simulink model "BodyModel_Simulink"  (R2020b)
settings: Solver=ode23tb  StartTime=0.0  StopTime=300  RelTol=1e-3
model workspace (MAT data in the model file):
  A_m = [-1000000  0  0  0  0  0  0  0  0  0  0  0; 0  -1000000  0  0  0  0  0  0  0  0  0  0; 0  0  -1000000  0  0  0  0  0  0  0  0  0; 0  0  0  -1000000  0  0  0  0  0  0  0  0; 0  0  0  0  -1000000  0  0  0  0  0  0  0; 0  0  0  0  0  -1000000  0  0  0  0  0  0; 0  0  0  0  0  0  -1000000  0  0  0  0  0; 0  0  0  0  0  0  0  -1000000  0  0  0  0; 0  0  0  0  0  0  0  0  -1000000  0  0  0; 0  0  0  0  0  0  0  0  0  -1000000  0  0; 0  0  0  0  0  0  0  0  0  0  -1000000  0; 0  0  0  0  0  0  0  0  0  0  0  -1000000]
  B_m = [1000000  0  0  0  0  0  0  0  0  0  0  0; 0  1000000  0  0  0  0  0  0  0  0  0  0; 0  0  1000000  0  0  0  0  0  0  0  0  0; 0  0  0  1000000  0  0  0  0  0  0  0  0; 0  0  0  0  1000000  0  0  0  0  0  0  0; 0  0  0  0  0  1000000  0  0  0  0  0  0; 0  0  0  0  0  0  1000000  0  0  0  0  0; 0  0  0  0  0  0  0  1000000  0  0  0  0; 0  0  0  0  0  0  0  0  1000000  0  0  0; 0  0  0  0  0  0  0  0  0  1000000  0  0; 0  0  0  0  0  0  0  0  0  0  1000000  0; 0  0  0  0  0  0  0  0  0  0  0  1000000]
  C_m = [1  0  0  0  0  0  0  0  0  0  0  0; 0  1  0  0  0  0  0  0  0  0  0  0; 0  0  1  0  0  0  0  0  0  0  0  0; 0  0  0  1  0  0  0  0  0  0  0  0; 0  0  0  0  1  0  0  0  0  0  0  0; 0  0  0  0  0  1  0  0  0  0  0  0; 0  0  0  0  0  0  1  0  0  0  0  0; 0  0  0  0  0  0  0  1  0  0  0  0; 0  0  0  0  0  0  0  0  1  0  0  0; 0  0  0  0  0  0  0  0  0  1  0  0; 0  0  0  0  0  0  0  0  0  0  1  0; 0  0  0  0  0  0  0  0  0  0  0  1]
  D_m = [0  0  0  0  0  0  0  0  0  0  0  0; 0  0  0  0  0  0  0  0  0  0  0  0; 0  0  0  0  0  0  0  0  0  0  0  0; 0  0  0  0  0  0  0  0  0  0  0  0; 0  0  0  0  0  0  0  0  0  0  0  0; 0  0  0  0  0  0  0  0  0  0  0  0; 0  0  0  0  0  0  0  0  0  0  0  0; 0  0  0  0  0  0  0  0  0  0  0  0; 0  0  0  0  0  0  0  0  0  0  0  0; 0  0  0  0  0  0  0  0  0  0  0  0; 0  0  0  0  0  0  0  0  0  0  0  0; 0  0  0  0  0  0  0  0  0  0  0  0]
  K_lqr = [0.500001142903  -0.499931060878  -0.5  1.16845749322  -1.17239239615  -5.45970154425  11.0305999607  10.9372947332  0.50006778687  5.97030096864  5.88033976668  5.40680902052; 0.499998857095  0.499931060724  -0.5  1.16845024596  1.17239040424  -5.45970154425  -11.0305542396  10.9372252078  -0.500070072517  -5.97026091208  5.88054448165  -5.40683381901; -0.499998857255  0.500068929772  -0.5  -1.16845223789  1.17271052724  -5.45970154425  -11.0320616409  -10.937270929  0.499932203623  -5.95555735243  -5.88058453821  5.40533797486; -0.500001142742  -0.500068929618  -0.5  -1.1684555013  -1.17270853533  -5.45970154425  11.0320159198  -10.937249012  -0.499929917976  5.95551729588  -5.88029971012  -5.40531317637]
  QuadrotorBodyModel_Object : BodyModel (value not decoded)
  ref_traj = timeseries
  ref_traj.Name = 'unnamed'
  ref_traj.DataInfo = tsdata.datametadata
  ref_traj.DataInfo.Interpolation = tsdata.interpolation
  ref_traj.DataInfo.Interpolation.Fhandle : function handle (value not decoded)
  ref_traj.DataInfo.Interpolation.Name = 'linear'
  ref_traj.TimeInfo = tsdata.timemetadata
  ref_traj.TimeInfo.Length = 619
  ref_traj.TimeInfo.DuplicateTimes = 0
  ref_traj.TimeInfo.Time_ = [0 0.01 0.02 0.03 0.04 0.05 0.06 0.07 0.08 0.09 0.1 0.11 ... (619 elements, 619x1)]
  ref_traj.TimeInfo.Initialized = 1
  ref_traj.QualityInfo = tsdata.qualmetadata
  ref_traj.Data_ = [0 0 0 0.0707113734695 -0.0707096056283 -0.000199998933321 0.141426919743 -0.141412775231 -0.000799982932534 0.212150815125 -0.212103067366 -0.00179991359088 ... (1857 elements, 3x1x619)]
  u_ss = [579.739564438; 579.739564438; 579.739564438; 579.739564438]
  x_des = [10; 10; -10; 0; 0; 0; 0; 0; 0; 0; 0; 0]
symbols that are objects in the model workspace (value not decoded): QuadrotorBodyModel_Object
libraries: uavutilslib x1
settings Model: OrderedModelArguments=off  Creator=prenk  LastModifiedBy=renkert2

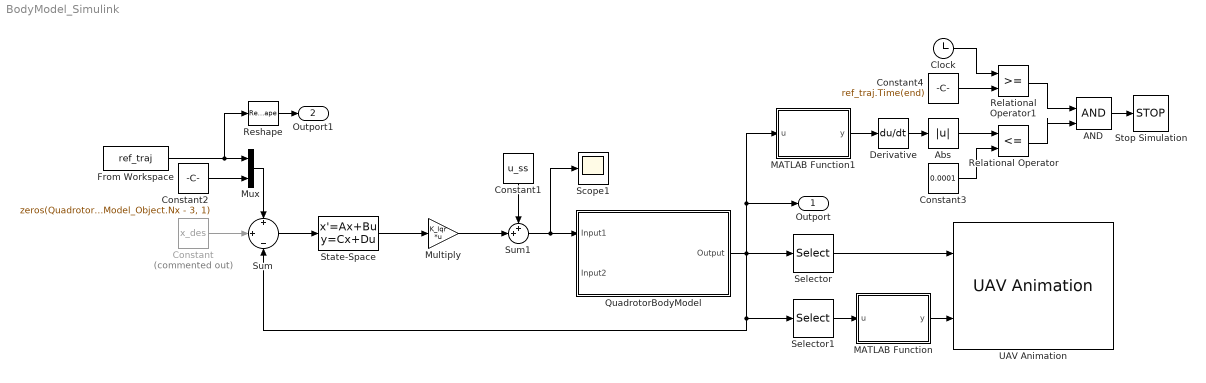
== system BodyModel_Simulink ==
  AND : Logic  IconShape=distinctive  AllPortsSameDT=off  OutDataTypeStr=boolean
  Abs : Abs
  Clock : Clock
  Constant : Constant  Commented=on  Value=x_des  VectorParams1D=off
  Constant1 : Constant  Value=u_ss  VectorParams1D=off
  Constant2 : Constant  Value=zeros(QuadrotorBodyModel_Object.Nx - 3, 1)
  Constant3 : Constant  Value=0.0001
  Constant4 : Constant  Value=ref_traj.Time(end)
  Derivative : Derivative  CoefficientInTFapproximation=100
  From Workspace : FromWorkspace  VariableName=ref_traj  OutputAfterFinalValue=Holding final value
  MATLAB Function : MATLAB Function  TreatAsAtomicUnit=on
  MATLAB Function1 : MATLAB Function  TreatAsAtomicUnit=on
  Multiply : Gain  Gain=K_lqr  Multiplication=Matrix(K*u)
  Mux : Mux  Inputs=2
  QuadrotorBodyModel : Subsystem  mask{x_0=[0;0;0;0;0;0;0;0;0;0;0;0]}
  Relational Operator : RelationalOperator  Operator=<=  OutDataTypeStr=boolean  RndMeth=Simplest
  Relational Operator1 : RelationalOperator  OutDataTypeStr=boolean  RndMeth=Simplest
  Reshape : Reshape
  Scope1 : Scope
  Selector : Selector  InputPortWidth=QuadrotorBodyModel_Object.Nx  IndexOptions=Index vector (dialog)  Indices=QuadrotorBodyModel_Object.I.x.p  OutputSizes=1
  Selector1 : Selector  InputPortWidth=QuadrotorBodyModel_Object.Nx  IndexOptions=Index vector (dialog)  Indices=QuadrotorBodyModel_Object.I.x.Theta  OutputSizes=1
  State-Space : StateSpace  A=A_m  B=B_m  C=C_m  D=D_m  InitialCondition=0
  Stop Simulation : Stop
  Sum : Sum  Inputs=+|+|-
  Sum1 : Sum  Inputs=++|
  UAV Animation : uavutilslib/UAV Animation  UAVType=Multirotor  UAVSize=1  InertialZDirection=Down  SampleTime=-1
      settings: SourceProductBaseCode=UV
  Outport : Outport  SignalName=y_out
  Outport1 : Outport  Port=2  SignalName=r_out
  wires:
  Constant/1 -> Sum/2
  Constant1/1 -> Sum1/1
  Sum1/1 -> Scope1/1, QuadrotorBodyModel/1(Input1)
  Multiply/1 -> Sum1/2
  Sum/1 -> State-Space/1
  State-Space/1 -> Multiply/1
  Mux/1 -> Sum/1
  Constant2/1 -> Mux/2
  Abs/1 -> Relational Operator/1
  Constant3/1 -> Relational Operator/2
  MATLAB Function1/1(y) -> Derivative/1
  Relational Operator/1 -> AND/2
  Clock/1 -> Relational Operator1/1
  Constant4/1 -> Relational Operator1/2
  Relational Operator1/1 -> AND/1
  AND/1 -> Stop Simulation/1
  Derivative/1 -> Abs/1
  From Workspace/1 -> Reshape/1, Mux/1
  Reshape/1 -> Outport1/1
  MATLAB Function/1(y) -> UAV Animation/2
  Selector1/1 -> MATLAB Function/1(u)
  Selector/1 -> UAV Animation/1
  QuadrotorBodyModel/1(Output) -> Selector1/1, Sum/3, Outport/1, MATLAB Function1/1(u), Selector/1

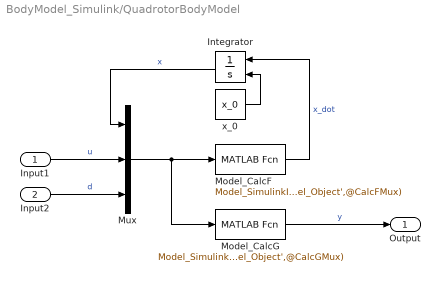
== system BodyModel_Simulink/QuadrotorBodyModel ==
  Input1 : Inport  PortDimensions=[QuadrotorBodyModel_Object.Nu,1]
  Input2 : Inport  Port=2
  Integrator : Integrator  InitialConditionSource=external
  Model_CalcF : MATLABFcn  MATLABFcn=Model_SimulinkInterpretedFunction(u,'BodyModel_Simulink','QuadrotorBodyModel_Object',@CalcFMux)  OutputDimensions=QuadrotorBodyModel_Object.Nx
  Model_CalcG : MATLABFcn  MATLABFcn=Model_SimulinkInterpretedFunction(u,'BodyModel_Simulink','QuadrotorBodyModel_Object',@CalcGMux)  OutputDimensions=QuadrotorBodyModel_Object.Ny
  Mux : Mux  Inputs=3
  x_0 : Constant  Value=x_0  VectorParams1D=off
  Output : Outport
  wires:
  Model_CalcF/1 -> Integrator/1  "x_dot"
  Input1/1 -> Mux/2  "u"
  Model_CalcG/1 -> Output/1  "y"
  x_0/1 -> Integrator/2
  Input2/1 -> Mux/3  "d"
  Integrator/1 -> Mux/1  "x"
  Mux/1 -> Model_CalcG/1, Model_CalcF/1

== matlab function BodyModel_Simulink/MATLAB Function ==
  data: u input; y output
function y = eul2quatMF(u)
    y = eul2quat([1 -1 1].*fliplr(u'),'ZYX');
end

== matlab function BodyModel_Simulink/MATLAB Function1 ==
  data: u input; y output
function y = vecnorm(u)

y = norm(u,2);
end
